simulink model "fir_filter_test_proj"  (R2019b)
settings: Solver=FixedStepDiscrete  StartTime=0.0  StopTime=0.0005  FixedStep=1e-6  RelTol=1e-3
libraries: aldec_ahdl x2, simulink_extras x1
settings Model: Creator=thomas  LastModifiedBy=thomas

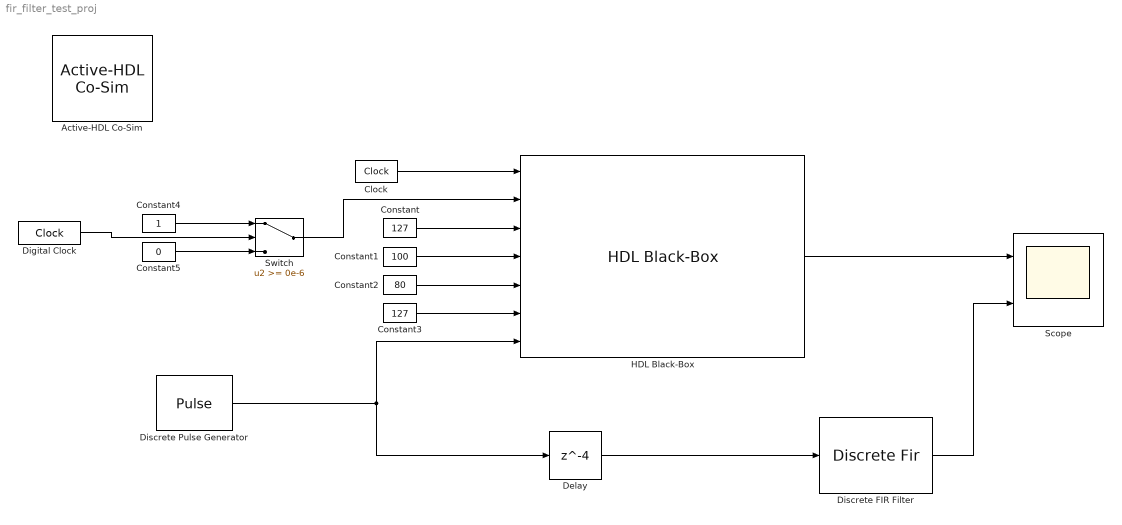
== system fir_filter_test_proj ==
  Active-HDL Co-Sim : aldec_ahdl/Active-HDL Co-Sim  Tag=Active-HDL_Co-Sim_close  hdl_period=1  hdl_tscale=us  sys_period=[1, 0]  sys_tscale=As In Simulator  wav_fn=$(model_name)  wav_settings=[0,3]  sim_cfg=[1,0,0]  dbg=off  auto_start=on  gen_tb=[0,1,15]  batch_sim=off  tb_fn=$(model_name).log  metavalue_map=[0,0]  sim_resolution=[1,0,1]  active_page=2  aws_en=off  ahdl_en=off  blk_ver=10.5a.RTM  macro_en=[0,0,0]
      settings: SourceProductName=Active-HDL Toolbox
  Clock : simulink_extras/Flip Flops/Clock  period=6e-6
  Constant : Constant  Value=127
  Constant1 : Constant  Value=100
  Constant2 : Constant  Value=80
  Constant3 : Constant  Value=127
  Constant4 : Constant
  Constant5 : Constant  Value=0
  Delay : Delay  DelayLength=4  InitialCondition=0  SampleTime=6e-6
  Digital Clock : DigitalClock  SampleTime=1e-6
  Discrete Pulse Generator : DiscretePulseGenerator  Amplitude=127  Period=10  SampleTime=6e-6
  Discrete FIR Filter : DiscreteFir  Coefficients=[127 100 80 127]  SampleTime=6e-6
  HDL Black-Box : aldec_ahdl/HDL Black-Box  Tag=Active-HDL_BB_lib  module_m=fir_filter_4  ports_cfg={i_clk,0,1,2,0,Inherited,8,0,0,0,0,1}{i_rstb,0,1,2,0,Inherited,8,0,0,0,0,1}{i_coeff_0,0,8,2,0,Inherited,0,0,0,0,0,1}{i_coeff_1,0,8,2,0,Inherited,0,0,0,0,0,1}{i_coeff_2,0,8,2,0,Inherited,0,0,0,0,0,1}{i_coeff_3,0,8,2,0,Inherited,0,0,0,0,0,1}{i_data,0,8,2,0,Inherited,0,0,0,0,0,1}{o_data,1,10,2,0,1,0,0,0,0,0,1}  waves={2,Inputs,2,3,0,15,,-1,-1,-1,0,0,0,0}{0,i_clk,0,0,0,15,,-1,-1,-1,0,0,0,0}{0,i_rstb,0,0,0,15,,-1,-1,-1,0,0,0,0}{0,i_coeff_0,2,2,0,15,,-1,-1,-1,1,0,0,0}{0,i_coeff_1,2,2,0,15,,-1,-1,-1,1,0,0,0}{0,i_coeff_2,2,2,0,15,,-1,-1,-1,1,0,0,0}{0,i_coeff_3,2,2,0,15,,-1,-1,-1,1,0,0,0}{0,i_data,2,2,0,15,,-1,-1,-1,1,0,0,0}{2,Outputs,2,3,0,15,,-1,-1,-1,0,0,0,0}{0,o_data,2,2,0,15,,-1,-1,-1,1,0,0,0}  block_mask=image('HDLBlackBox.jpg','center'); disp('fir_filter_4');port_label('input', 1, 'i_clk');port_label('input', 2, 'i_rstb');port_label('input', 3, 'i_coeff_0');port_label('input', 4, 'i_coeff_1');port_label('input', 5, 'i_coeff_2');port_label('input', 6, 'i_coeff_3');port_label('input', 7, 'i_data');port_label('output', 1, 'o_data');  config=[7,1]  inp=[7, 8, 1, 0, 0, 0, 2, 8, 1, 0, 0, 0, 2, 0, 8, 0, 0, 0, 2, 0, 8, 0, 0, 0, 2, 0, 8, 0, 0, 0, 2, 0, 8, 0, 0, 0, 2, 0, 8, 0, 0, 0, 2]  out=[1, 0, 10, 0, 0, 0, 2]  sampling=[1, -1, -1, -1, -1, -1, -1, -1, 1]  active_page={766,476,0,{0,{80,0,0,1},{35,1,2,1},{65,2,2,1},{70,3,2,1},{70,4,2,1},{60,5,2,1},{60,6,2,1},{50,7,2,1},{35,8,2,1},{36,9,2,1},{119,10,0,1}},{1,{106,0,0,1},{55,1,2,1},{70,2,2,1},{75,3,2,1},{75,4,2,1},{45,5,2,1},{45,6,2,1},{45,7,2,1},{165,8,0,1}},{2,{165,0,0,1},{130,1,2,1},{190,2,2,1},{190,3,2,1}},{3,{94,0,0,1},{58,1,2,1},{58,2,2,1},{70,3,2,1},{58,4,2,1}},{4,{83,0,0,1},{70,1,2,1},{80,2,2,1},{50,3,2,1},{50,4,2,1}},{5,{125,0,0,1},{330,1,2,1},{220,2,2,1}},{6,{95,0,0,1},{95,1,1,1},{70,2,2,1},{50,3,1,1},{80,4,1,1},{35,5,2,1},{35,6,2,1},{65,7,0,1},{150,8,0,1}}}  param_val=0  clk_val=[0]  ce_val=[0]  blk_ver=10.5a.RTM  blk_conf=0  user_conv=0
      settings: SourceProductName=Active-HDL Toolbox
  Scope : Scope  NumInputPorts=2
  Switch : Switch  Threshold=0e-6
  wires:
  Constant/1 -> HDL Black-Box/3
  Constant3/1 -> HDL Black-Box/6
  Constant2/1 -> HDL Black-Box/5
  Constant1/1 -> HDL Black-Box/4
  Clock/1 -> HDL Black-Box/1
  HDL Black-Box/1 -> Scope/1
  Discrete FIR Filter/1 -> Scope/2
  Switch/1 -> HDL Black-Box/2
  Constant4/1 -> Switch/1
  Constant5/1 -> Switch/3
  Digital Clock/1 -> Switch/2
  Discrete Pulse Generator/1 -> Delay/1, HDL Black-Box/7
  Delay/1 -> Discrete FIR Filter/1
